simulink model "stellaris_test_pilcov"  (R2013a)
settings: Solver=FixedStepDiscrete  StartTime=0.0  StopTime=inf  FixedStep=0.1  RelTol=1e-3
settings Model: Creator=peselnikmg  LastModifiedBy=peselnikmg
settings OptimizationCC: ExpressionDepthLimit=2147483647  OptimizeModelRefInitCode=on  LifeSpan=1
settings DebuggingCC: UnderspecifiedInitializationDetection=Simplified  MergeDetectMultiDrivingBlocksExec=error  StrictBusMsg=ErrorOnBusTreatedAsVector  NonBusSignalsTreatedAsBus=error
settings HardwareCC: ProdEndianess=LittleEndian  ProdHWDeviceType=Texas Instruments->TMS470
settings RTWCC: SystemTargetFile=stellaris.tlc  TemplateMakefile=stellaris_tmf  PostCodeGenCommand=stellaris_customcode(buildInfo)  Description=TI Stellaris LaunchPad  ProcessScript=stellaris_make_rtw_hook
settings CodeAppCC: IgnoreCustomStorageClasses=off  CustomSymbolStrType=$N$R$M
settings STFCustomTargetCC: CombineOutputUpdateFcns=on  ERTCustomFileBanners=on  SupportContinuousTime=off  SupportNonInlinedSFcns=off  MATLABClassNameForMDSCustomization=Simulink.SoftwareTarget.ERTCustomization  SystemTargetFile=stellaris.tlc
settings ERTTargetCC: GenerateSampleERTMain=off  ParMdlRefBuildCompliant=off  CompOptLevelCompliant=off  ConcurrentExecutionCompliant=off  ERTFirstTimeCompliant=off  ModelStepFunctionPrototypeControlCompliant=off  CPPClassGenCompliant=off  ERTCustomFileTemplate=stellaris_srmain.tlc

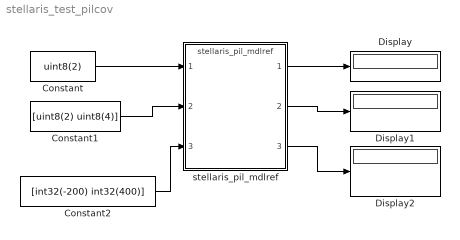
== system stellaris_test_pilcov ==
  Constant : Constant  Value=uint8(2)  SampleTime=0.1
  Constant1 : Constant  Value=[uint8(2) uint8(4)]  SampleTime=0.1
  Constant2 : Constant  Value=[int32(-200) int32(400)]  SampleTime=0.1
  Display : Display
  Display1 : Display
  Display2 : Display
  stellaris_pil_mdlref : ModelReference  ModelNameDialog=stellaris_pil_mdlref  SimulationMode=Processor-in-the-loop (PIL)  ModelReferenceVersion=1.15  CopyOfModelName=stellaris_pil_mdlref  DefaultDataLogging=on
  wires:
  stellaris_pil_mdlref/1 -> Display/1
  Constant/1 -> stellaris_pil_mdlref/1
  Constant1/1 -> stellaris_pil_mdlref/2
  stellaris_pil_mdlref/2 -> Display1/1
  stellaris_pil_mdlref/3 -> Display2/1
  Constant2/1 -> stellaris_pil_mdlref/3
